simulink model "inelastic_single"  (R2018b)
settings: Solver=VariableStepAuto  StartTime=0.0  StopTime=10.0  RelTol=1e-3
values from neighbouring files (symbols this model uses):
  seed = 1    [Network_configuration.m]
undefined symbols (not defined in the file or in its folder): m, n
libraries: simulink x2
settings Model: Creator=Jiaxiao Zheng  LastModifiedBy=Jiaxiao Zheng

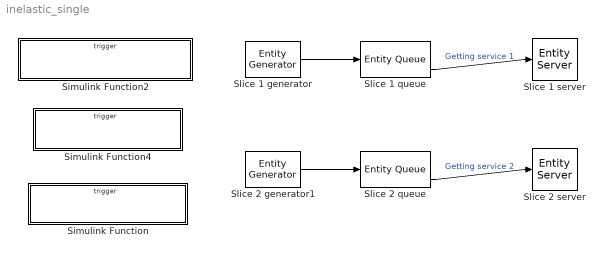
== system inelastic_single ==
  " Slice 1 server" : EntityServer  InputPortMessageModes=m  OutputPortMessageModes=m  Capacity=50  ServiceTimeValue=0  EntryAction=|
      | assert(size(entity.Id, 1) == 1);
      | assert(size(entity.Id, 2) == 1);
      | assert(entity.Slice == 1);
      | [entity.arrival, entity.socketId] = serving(-1, ...
      |     entity.ServiceTime, 1, entity.Type, 1);
  " Slice 2 server" : EntityServer  InputPortMessageModes=m  OutputPortMessageModes=m  Capacity=50  ServiceTimeValue=0  EntryAction=|
      | assert(size(entity.Id, 1) == 1);
      | assert(size(entity.Id, 2) == 1);
      | assert(entity.Slice == 2);
      | [entity.arrival, entity.socketId] = serving(-1, ...
      |     entity.ServiceTime, 2, entity.Type, 1);
  Simulink Function : Subsystem  TreatAsAtomicUnit=on
  Simulink Function2 : Subsystem  TreatAsAtomicUnit=on
  Simulink Function4 : Subsystem  TreatAsAtomicUnit=on
  Slice 1 generator : EntityGenerator  OutputPortMessageModes=m  TimeSource=MATLAB action  IntergenerationTimeAction=dt = exponentialArrivalTime(1);  GenerateEntityAtSimulationStart=off  GenerateAction=|  AttributeName=ServiceTime|Id|Slice|Type|arrival|departure|socketId  AttributeInitialValue=1|1|1|1|0|0|-1  EntityType=Structured  EntityTypeName=Entity
      | entity.ServiceTime = serviceTime(1);
      | entity.Id = idAllocation();
  Slice 1 queue : EntityQueue  InputPortMessageModes=m  OutputPortMessageModes=n,m  Capacity=10000  NumberEntitiesDeparted=on
      settings: OutputPortMap=o0,o5
  Slice 2 generator1 : EntityGenerator  OutputPortMessageModes=m  TimeSource=MATLAB action  IntergenerationTimeAction=dt = exponentialArrivalTime(1);  GenerateEntityAtSimulationStart=off  GenerateAction=|  AttributeName=ServiceTime|Id|Slice|Type|arrival|departure|socketId  AttributeInitialValue=1|1|1|1|0|0|-1  EntityType=Structured  EntityTypeName=Entity
      | entity.ServiceTime = serviceTime(1);
      | entity.Id = idAllocation();
  Slice 2 queue : EntityQueue  InputPortMessageModes=m  OutputPortMessageModes=n,m  Capacity=10000  NumberEntitiesDeparted=on
      settings: OutputPortMap=o0,o5
  wires:
  Slice 1 generator/1 -> Slice 1 queue/1
  Slice 2 generator1/1 -> Slice 2 queue/1
  Slice 1 queue/2 -> " Slice 1 server"/1  "Getting service 1"
  Slice 2 queue/2 -> " Slice 2 server"/1  "Getting service 2"

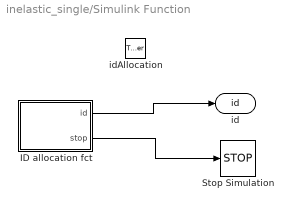
== system inelastic_single/Simulink Function ==
  idAllocation : TriggerPort  TriggerType=function-call  IsSimulinkFunction=on  FunctionName=idAllocation  VariantControl=(inherit)
  " ID allocation fct" : MATLAB Function  TreatAsAtomicUnit=on
  Stop Simulation : Stop
  id : ArgOut  DisableCoverage=on  ArgumentName=id
  wires:
  " ID allocation fct"/1(id) -> id/1
  " ID allocation fct"/2(stop) -> Stop Simulation/1

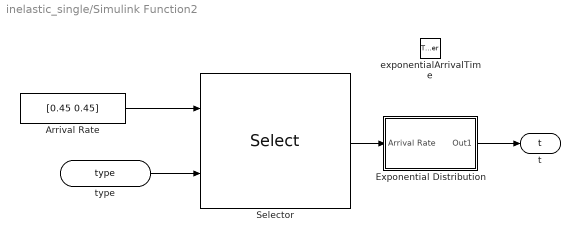
== system inelastic_single/Simulink Function2 ==
  exponentialArrivalTime : TriggerPort  TriggerType=function-call  IsSimulinkFunction=on  FunctionName=exponentialArrivalTime  VariantControl=Variant
  Arrival Rate : Constant  Value=[0.45 0.45]  SampleTime=-1
  Exponential Distribution : Subsystem
  Selector : Selector  IndexOptions=Index vector (port)  Indices=[1 3]  OutputSizes=1
  type : ArgIn  DisableCoverage=on  ArgumentName=type
  t : ArgOut  DisableCoverage=on  ArgumentName=t
  wires:
  Exponential Distribution/1(Out1) -> t/1
  Arrival Rate/1 -> Selector/1
  Selector/1 -> Exponential Distribution/1(Arrival Rate)
  type/1 -> Selector/2

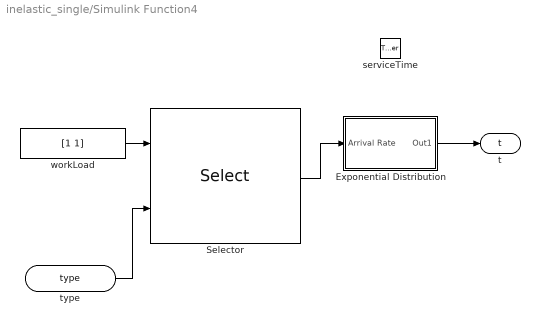
== system inelastic_single/Simulink Function4 ==
  serviceTime : TriggerPort  TriggerType=function-call  IsSimulinkFunction=on  FunctionName=serviceTime  VariantControl=Variant
  Exponential Distribution : Subsystem
  Selector : Selector  IndexOptions=Index vector (port)  Indices=[1 3]  OutputSizes=1
  workLoad : Constant  Value=[1 1]  SampleTime=-1
  type : ArgIn  DisableCoverage=on  ArgumentName=type
  t : ArgOut  DisableCoverage=on  ArgumentName=t
  wires:
  Exponential Distribution/1(Out1) -> t/1
  type/1 -> Selector/2
  workLoad/1 -> Selector/1
  Selector/1 -> Exponential Distribution/1(Arrival Rate)

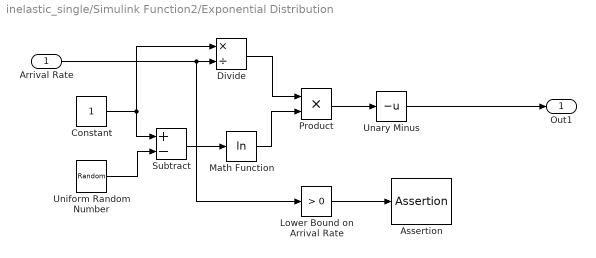
== system inelastic_single/Simulink Function2/Exponential Distribution ==
  Arrival Rate : Inport
  Assertion : Assertion
  Constant : Constant
  Divide : Product  Inputs=*/
  Lower Bound on Arrival Rate : simulink/Logic and Bit Operations/Compare To Constant  relop=>  const=0  OutDataTypeStr=uint8  ZeroCross=off
  Math Function : Math  Operator=log  SaturateOnIntegerOverflow=on
  Product : Product  RndMeth=Zero
  Subtract : Sum  Inputs=+-
  Unary Minus : UnaryMinus
  Uniform Random Number : UniformRandomNumber  Minimum=0  Seed=seed
  Out1 : Outport
  wires:
  Subtract/1 -> Math Function/1
  Lower Bound on Arrival Rate/1 -> Assertion/1
  Uniform Random Number/1 -> Subtract/2
  Constant/1 -> Subtract/1, Divide/1
  Divide/1 -> Product/1
  Math Function/1 -> Product/2
  Product/1 -> Unary Minus/1
  Unary Minus/1 -> Out1/1
  Arrival Rate/1 -> Lower Bound on Arrival Rate/1, Divide/2

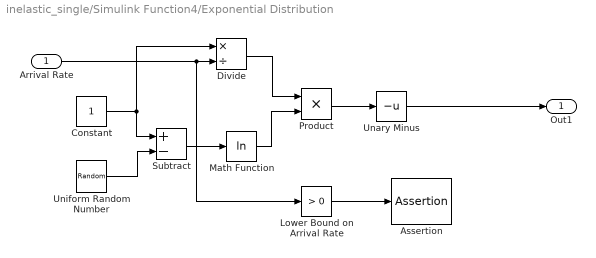
== system inelastic_single/Simulink Function4/Exponential Distribution ==
  Arrival Rate : Inport
  Assertion : Assertion
  Constant : Constant
  Divide : Product  Inputs=*/
  Lower Bound on Arrival Rate : simulink/Logic and Bit Operations/Compare To Constant  relop=>  const=0  OutDataTypeStr=uint8  ZeroCross=off
  Math Function : Math  Operator=log  SaturateOnIntegerOverflow=on
  Product : Product  RndMeth=Zero
  Subtract : Sum  Inputs=+-
  Unary Minus : UnaryMinus
  Uniform Random Number : UniformRandomNumber  Minimum=0  Seed=12345
  Out1 : Outport
  wires:
  Subtract/1 -> Math Function/1
  Lower Bound on Arrival Rate/1 -> Assertion/1
  Uniform Random Number/1 -> Subtract/2
  Constant/1 -> Subtract/1, Divide/1
  Divide/1 -> Product/1
  Math Function/1 -> Product/2
  Product/1 -> Unary Minus/1
  Unary Minus/1 -> Out1/1
  Arrival Rate/1 -> Lower Bound on Arrival Rate/1, Divide/2

== matlab function inelastic_single/Simulink Function/ ID allocation fct ==
  data: id output; stop output
function [id, stop] = fcn
persistent userCnt;
if isempty(userCnt)
    userCnt = 0;
end
userCnt = userCnt + 1;
id = userCnt;
%stop = (id >= 1000);
stop = 0;
